simulink model "SIR"  (R2020b)
settings: Solver=VariableStepAuto  StartTime=0.0  StopTime=200  RelTol=1e-3
undefined symbols (not defined in the file or in its folder): parSIR
settings Model: Creator=parze  LastModifiedBy=Simon

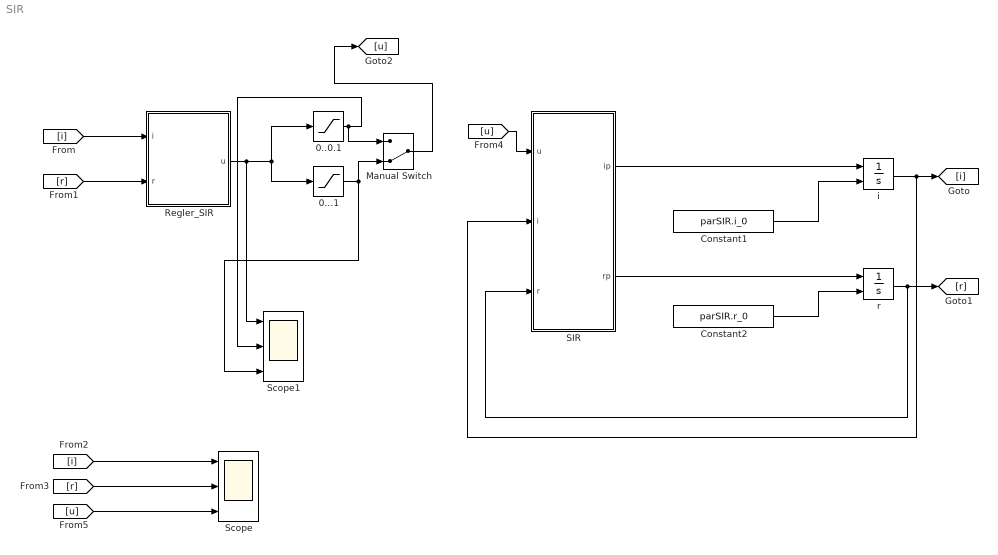
== system SIR ==
  0...1 : Saturate  UpperLimit=1  LowerLimit=0
  0..0.1 : Saturate  UpperLimit=0.1  LowerLimit=0
  Constant1 : Constant  Value=parSIR.i_0
  Constant2 : Constant  Value=parSIR.r_0
  Manual Switch : ManualSwitch  CurrentSetting=0
  Regler_SIR : MATLAB Function  TreatAsAtomicUnit=on
  SIR : MATLAB Function  TreatAsAtomicUnit=on
  Scope : Scope  NumInputPorts=3
  Scope1 : Scope  NumInputPorts=3
  i : Integrator  InitialConditionSource=external
  r : Integrator  InitialConditionSource=external
  wires:
  SIR/1(ip) -> i/1
  SIR/2(rp) -> r/1
  i/1 -> SIR/2(i), [i]
  r/1 -> SIR/3(r), [r]
  [i] -> Regler_SIR/1(i)
  [r] -> Regler_SIR/2(r)
  Constant1/1 -> i/2
  [r] -> Scope/2
  [i] -> Scope/1
  Constant2/1 -> r/2
  [u] -> SIR/1(u)
  [u] -> Scope/3
  Manual Switch/1 -> [u]
  0..0.1/1 -> Scope1/2, Manual Switch/1
  0...1/1 -> Scope1/3, Manual Switch/2
  Regler_SIR/1(u) -> 0..0.1/1, 0...1/1, Scope1/1

== matlab function SIR/SIR ==
  settings: updateMethod=CONTINUOUS
  data: u input; i input; r input; ip output; parSIR parameter; rp output
function [ip,rp]= SIR(u,i,r,parSIR)
   
    beta = parSIR.beta
    gamma = parSIR.gamma
    delta = parSIR.delta

    ip =  beta.*i.*(1-i-r) - gamma.*i;
    rp = gamma.*i - delta.*r + u;

== matlab function SIR/Regler_SIR ==
  settings: updateMethod=CONTINUOUS
  data: i input; r input; u output; parSIR parameter
function u = Regler(i,r,parSIR)

c1=0.1;
c2=1;

% ohne Beschränkung
%     c1=2;
%     c2=4;

% mit Beschränkung
%     c1=0.1;
%     c2=1;

beta = parSIR.beta;
gamma_ = parSIR.gamma;
delta = parSIR.delta;
i_soll = parSIR.i_soll;

u = (0.2e1 * i ^ 2 * (i + r / 0.2e1 - i_soll / 0.2e1 - 0.1e1 / 0.2e1) * beta ^ 2 + (-i ^ 2 * c2 + (-c1 * i_soll + (-r + 0.1e1) * c2 + delta * r) * i - c1 * i_soll * (r - 0.1e1)) * beta + c2 * (c1 - gamma_) * i - c1 * i_soll * (c2 + gamma_)) / i / beta;
